simulink model "TP1_Hacheur_serie"  (R2024a)
settings: Solver=ode45  StartTime=0.0  StopTime=0.3  MaxStep=1e-3  RelTol=1e-4
values from neighbouring files (symbols this model uses):
  alpha = 25    [TP_Hacheurs.m]
  E = 0    [TP_Hacheurs.m]
  L = 0.1    [TP_Hacheurs.m]
  R = 10    [TP_Hacheurs.m]
  T = 1/f    (= 0.002)    [TP_Hacheurs.m]
  Vdc = 50    [TP_Hacheurs.m]
libraries: spsCurrentMeasurementLib x3, spsMeanPhasorLib x2, spsDCVoltageSourceLib x2, spsDiodeLib x1, spsIGBTDiodeLib x1, spsSeriesRLCBranchLib x1, spsVoltageMeasurementLib x1, sps_lib x1
settings Model: Creator=Legrey  LastModifiedBy=macbookair
settings DataIOCC: ReturnWorkspaceOutputs=off
settings RTWCC: GPUComputeCapability=3.5

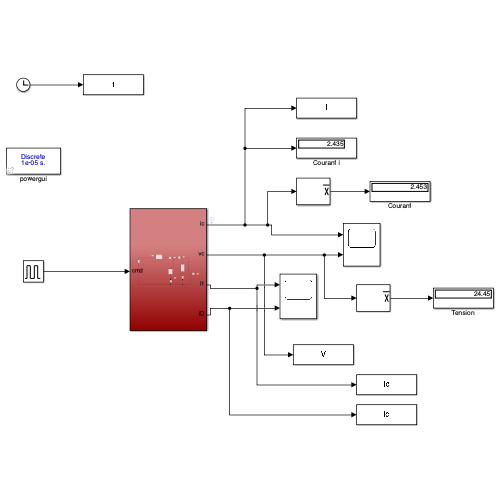
[thumbnail: Simulink's stored preview of the top-level diagram]
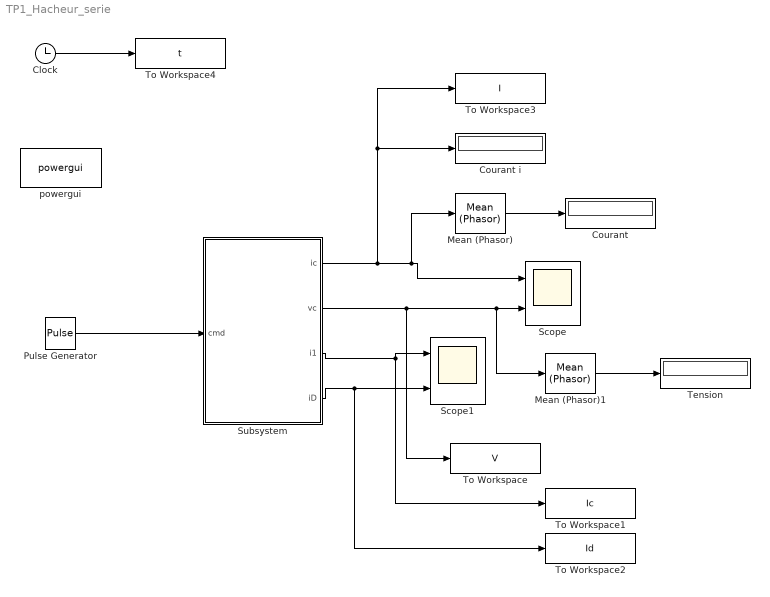
== system TP1_Hacheur_serie ==
  Clock : Clock
  Courant : Display
  Courant i : Display
  Mean (Phasor) : spsMeanPhasorLib/Mean (Phasor)  Freq=f  Vinit=0  Ts=0
      settings: LibrarySourceBlock=|
      | sps_lib/Sensors and Measurements/Mean
      | (Phasor)
  Mean (Phasor)1 : spsMeanPhasorLib/Mean (Phasor)  Freq=f  Vinit=0  Ts=0
      settings: LibrarySourceBlock=|
      | sps_lib/Sensors and Measurements/Mean
      | (Phasor)
  Pulse Generator : DiscretePulseGenerator  PulseType=Time based  Period=T  PulseWidth=alpha
  Scope : Scope  NumInputPorts=2
  Scope1 : Scope  NumInputPorts=2
  Subsystem : Subsystem
  Tension : Display
  To Workspace : ToWorkspace  VariableName=V  SampleTime=-1
  To Workspace1 : ToWorkspace  VariableName=Ic  SampleTime=-1
  To Workspace2 : ToWorkspace  VariableName=Id  SampleTime=-1
  To Workspace3 : ToWorkspace  VariableName=I  SampleTime=-1
  To Workspace4 : ToWorkspace  VariableName=t  SampleTime=-1
  powergui : sps_lib/powergui  Priority=1  SimulationMode=Discrete  SampleTime=1e-005  frequency=60  Iterations=50  frequencyindice=0  Pbase=100e6  ErrMax=1e-4  UnitsV=kV  UnitsW=MW  buscounter=0  FunctionMessages=off  echomessages=off  EnableUseOfTLC=off  CurrentSourceSwitches=off  DisableSnubberDevices=off  DisableRonSwitches=off  DisableVfSwitches=off  DisplayEquations=off  AutomaticDiscreteSolvers=off  SolverType=Tustin/Backward Euler (TBE)  Interpol=off  ExternalGateDelay=off  methode=off  Ts=100  x0status=blocks  SPID=on  SwTol=0  HookPort=off  NonlinearTolerance=1e-4  nMaxIteration=100  ContinueOnMaxIteration=off  RestoreLinks=warning  ResistiveCurrentMeasurement=off  Frange=[0:2:500]  Ylog=off  Xlog=on  ShowGrid=off  save=off  variable=ZData  structure=0  ZoomFFT=off  StartTime=0.0  cycles=1  DisplayStyle=1  fundamental=60  FreqAxis=off  MaxFrequency=1000  frequencyindicesteady=1  RmsSteady=1  display=off
  wires:
  Pulse Generator/1 -> Subsystem/1(cmd)
  Subsystem/1(ic) -> To Workspace3/1, Courant i/1, Mean (Phasor)/1, Scope/1
  Subsystem/2(vc) -> To Workspace/1, Mean (Phasor)1/1, Scope/2
  Subsystem/3(i1) -> To Workspace1/1, Scope1/1
  Subsystem/4(iD) -> To Workspace2/1, Scope1/2
  Mean (Phasor)/1 -> Courant/1
  Mean (Phasor)1/1 -> Tension/1
  Clock/1 -> To Workspace4/1

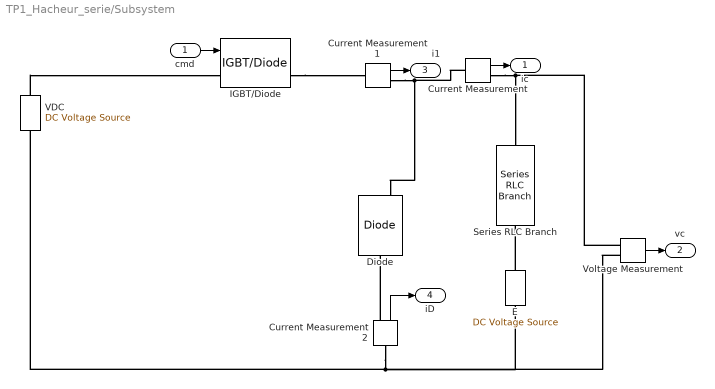
== system TP1_Hacheur_serie/Subsystem ==
  cmd : Inport
  Current Measurement : spsCurrentMeasurementLib/Current Measurement  PhasorSimulation=off  OutputType=Complex  PSBequivalent=0
  Current Measurement1 : spsCurrentMeasurementLib/Current Measurement  PhasorSimulation=off  OutputType=Complex  PSBequivalent=0
  Current Measurement2 : spsCurrentMeasurementLib/Current Measurement  PhasorSimulation=off  OutputType=Complex  PSBequivalent=0
  Diode : spsDiodeLib/Diode  Ron=0.001  Lon=0  Vf=0.8  IC=0  UseSnubber=0  Rs=500  Cs=250e-9  Measurements=on
  E : spsDCVoltageSourceLib/DC Voltage Source  Amplitude=E  Measurements=None
  IGBT/Diode : spsIGBTDiodeLib/IGBT//Diode  Ron=1e-3  Rs=1e5  Cs=inf  Measurements=on
  Series RLC Branch : spsSeriesRLCBranchLib/Series RLC Branch  LConnTagsString=__new0  RConnTagsString=__new0  BranchType=RL  Resistance=R  Inductance=L  SetiL0=off  InitialCurrent=0  Capacitance=0  Setx0=off  InitialVoltage=0  Measurements=None
  VDC : spsDCVoltageSourceLib/DC Voltage Source  Amplitude=Vdc  Measurements=None
  Voltage Measurement : spsVoltageMeasurementLib/Voltage Measurement  PhasorSimulation=off  OutputType=Complex  PSBequivalent=0
  ic : Outport
  vc : Outport  Port=2
  i1 : Outport  Port=3
  iD : Outport  Port=4
  wires:
  cmd/1 -> IGBT/Diode/1
  Voltage Measurement/1 -> vc/1
  Current Measurement/1 -> ic/1
  Current Measurement1/1 -> i1/1
  Current Measurement2/1 -> iD/1
  connections:
  Current Measurement1/RConn1 -- Diode/RConn1 -- Current Measurement/LConn1
  Current Measurement/RConn1 -- Series RLC Branch/LConn1 -- Voltage Measurement/LConn1
  Current Measurement2/LConn1 -- Voltage Measurement/LConn2 -- E/LConn1 -- VDC/LConn1
  E/RConn1 -- Series RLC Branch/RConn1
  VDC/RConn1 -- IGBT/Diode/LConn1
  IGBT/Diode/RConn1 -- Current Measurement1/LConn1
  Current Measurement2/RConn1 -- Diode/LConn1
